simulink model "RobotControl"  (R2016a)
settings: Solver=FixedStepDiscrete  StartTime=0.0  StopTime=16  FixedStep=0.005  RelTol=1e-3
values from neighbouring files (symbols this model uses):
  BACKWARD = 2    [ControlInit.m]
  BUSY = 4    [ControlInit.m]
  CCW = 4    [ControlInit.m]
  CLEANED = 2    [ControlInit.m]
  CW = 3    [ControlInit.m]
  EMPTY = 3    [ControlInit.m]
  FORWARD = 1    [ControlInit.m]
  GTSP = 25    [ControlInit.m]
  initX = uint8((ROOM_SIDE_SIZE/2) - 1)    [ControlInit.m]
  initY = initX    [ControlInit.m]
  LEFT_BUSY_RIGHT_BUSY = 9    [ControlInit.m]
  LEFT_BUSY_RIGHT_CLEANED = 14    [ControlInit.m]
  LEFT_BUSY_RIGHT_EMPTY = 7    [ControlInit.m]
  LEFT_CLEANED_RIGHT_BUSY = 13    [ControlInit.m]
  LEFT_CLEANED_RIGHT_CLEANED = 12    [ControlInit.m]
  LEFT_CLEANED_RIGHT_EMPTY = 10    [ControlInit.m]
  LEFT_EMPTY_RIGHT_BUSY = 8    [ControlInit.m]
  LEFT_EMPTY_RIGHT_CLEANED = 11    [ControlInit.m]
  LEFT_EMPTY_RIGHT_EMPTY = 15    [ControlInit.m]
  map = uint8(ones(ROOM_SIDE_SIZE , ROOM_SIDE_SIZE)*UNCOVERED)    [ControlInit.m]
  MOVE_TURN_LEFT = 20    [ControlInit.m]
  MOVE_TURN_RIGHT = 21    [ControlInit.m]
  MOVE_U_TURN = 24    [ControlInit.m]
  MOVE_U_TURN_LEFT = 23    [ControlInit.m]
  MOVE_U_TURN_RIGHT = 22    [ControlInit.m]
  ROB_EAST = 0    [ControlInit.m]
  ROB_ERRVAL = 5    [ControlInit.m]
  ROB_NONE = 400    [ControlInit.m]
  ROB_NORTH = 270    [ControlInit.m]
  ROB_SOUTH = 90    [ControlInit.m]
  ROB_WEST = 180    [ControlInit.m]
  ROOM_SIDE_SIZE = 20    [ControlInit.m]
  STOP = 5    [ControlInit.m]
  UNCOVERED = 1    [ControlInit.m]
  ZIGZAG = 26    [ControlInit.m]
undefined symbols (not defined in the file or in its folder): COMH, Compass_Handler, MovementHandler, MOVH, POSH, positionHandler, ROB_LENG, ROTH, Routines, SAMPLE_TIME
libraries: simulink x2, SCAN x1, MAPH x1, MOTH x1
(part 2 of 2)

== stateflow chart RobotControl/Routines/HitSensorViewCalculation/pumperHitSensorView ==
  state SensorViewState
  state Init
    entry:
    sensorView = 0;
  state NoHit
    entry:
    currentY = c_Y - 1;
    currentX = c_X - 1;
  (junction 10) -> SensorViewState [order 1] : [(map[currentY][currentX - 1] == BUSY) ...
      | && ( (map[currentY][currentX + 1] == EMPTY)...
      |  || (map[currentY][currentX+1] == UNCOVERED) )]...
      | /sensorView = LEFT_BUSY_RIGHT_EMPTY;
  (junction 10) -> SensorViewState [order 2] : [(map[currentY][currentX - 1] == CLEANED) ...
      | && ((map[currentY][currentX + 1] == EMPTY)...
      | || (map[currentY][currentX+1] == UNCOVERED))]
      | /{sensorView =  LEFT_CLEANED_RIGHT_EMPTY;}
  (junction 10) -> SensorViewState [order 3] : [((map[currentY][currentX - 1] == EMPTY) ...
      | || (map[currentY][currentX - 1] == UNCOVERED))...
      | && (map[currentY][currentX + 1] == BUSY)]
      | /{sensorView = LEFT_EMPTY_RIGHT_BUSY;}
  (junction 10) -> SensorViewState [order 4] : [(map[currentY][currentX + 1] == CLEANED) ...
      | && ((map[currentY][currentX - 1] == EMPTY)...
      | || (map[currentY][currentX - 1] == UNCOVERED))]
      | /{sensorView =  LEFT_EMPTY_RIGHT_CLEANED;}
  (junction 10) -> SensorViewState [order 5] : [((map[currentY][currentX + 1] == EMPTY) ...
      | || (map[currentY][currentX + 1] == UNCOVERED))...
      | && ((map[currentY][currentX - 1] == EMPTY)...
      | || (map[currentY][currentX - 1] == UNCOVERED))]
      | /{sensorView = LEFT_EMPTY_RIGHT_EMPTY;}
  (junction 10) -> SensorViewState [order 6] : [(map[currentY][currentX - 1] == BUSY) ...
      | && (map[currentY][currentX + 1] == BUSY)]
      | /{sensorView = LEFT_BUSY_RIGHT_BUSY;}
  (junction 10) -> SensorViewState [order 7] : [(map[currentY][currentX - 1] == CLEANED) ...
      | && (map[currentY][currentX + 1] == CLEANED)]
      | /{sensorView = LEFT_CLEANED_RIGHT_CLEANED;}
  (junction 10) -> SensorViewState [order 8] : [(map[currentY][currentX - 1] == BUSY) ...
      | && (map[currentY][currentX + 1] == CLEANED)]
      | /{sensorView = LEFT_BUSY_RIGHT_CLEANED;}
  (junction 10) -> SensorViewState [order 9] : [(map[currentY][currentX - 1] == CLEANED) ...
      | && (map[currentY][currentX + 1] == BUSY)]
      | /{sensorView = LEFT_CLEANED_RIGHT_BUSY;}
  (junction 8) -> (junction 10) [order 1] : [currentHeading == ROB_NORTH]
  (default) -> Init
  (junction 11) -> SensorViewState [order 2] : [(map[currentY][currentX - 1] == BUSY) ...
      | && ( (map[currentY][currentX + 1] == EMPTY)...
      |  || (map[currentY][currentX+1] == UNCOVERED) )]...
      | /sensorView = LEFT_EMPTY_RIGHT_BUSY;
  Init -> NoHit
  NoHit -> (junction 8) : [pumperHit_BOOL]
  (junction 8) -> (junction 15) [order 4] : [currentHeading == ROB_EAST]
  (junction 8) -> (junction 13) [order 3] : [currentHeading == ROB_WEST]
  (junction 8) -> (junction 11) [order 2] : [currentHeading == ROB_SOUTH]
  SensorViewState -> NoHit
  (junction 11) -> SensorViewState [order 1] : [(map[currentY][currentX - 1] == CLEANED) ...
      | && ((map[currentY][currentX + 1] == EMPTY)...
      | || (map[currentY][currentX+1] == UNCOVERED))]
      | /{sensorView =  LEFT_EMPTY_RIGHT_CLEANED;}
  (junction 11) -> SensorViewState [order 5] : [((map[currentY][currentX - 1] == EMPTY) ...
      | || (map[currentY][currentX - 1] == UNCOVERED))...
      | && (map[currentY][currentX + 1] == BUSY)]
      | /{sensorView = LEFT_BUSY_RIGHT_EMPTY;}
  (junction 11) -> SensorViewState [order 6] : [(map[currentY][currentX + 1] == CLEANED) ...
      | && ((map[currentY][currentX - 1] == EMPTY)...
      | || (map[currentY][currentX - 1] == UNCOVERED))]
      | /{sensorView =  LEFT_CLEANED_RIGHT_EMPTY;}
  (junction 11) -> SensorViewState [order 4] : [((map[currentY][currentX + 1] == EMPTY) ...
      | || (map[currentY][currentX + 1] == UNCOVERED))...
      | && ((map[currentY][currentX - 1] == EMPTY)...
      | || (map[currentY][currentX - 1] == UNCOVERED))]
      | /{sensorView = LEFT_EMPTY_RIGHT_EMPTY;}
  (junction 11) -> SensorViewState [order 8] : [(map[currentY][currentX - 1] == BUSY) ...
      | && (map[currentY][currentX + 1] == CLEANED)]
      | /{sensorView = LEFT_CLEANED_RIGHT_BUSY;}
  (junction 11) -> SensorViewState [order 3] : [(map[currentY][currentX - 1] == BUSY) ...
      | && (map[currentY][currentX + 1] == BUSY)]
      | /{sensorView = LEFT_BUSY_RIGHT_BUSY;}
  (junction 11) -> SensorViewState [order 7] : [(map[currentY][currentX - 1] == CLEANED) ...
      | && (map[currentY][currentX + 1] == CLEANED)]
      | /{sensorView = LEFT_CLEANED_RIGHT_CLEANED;}
  (junction 11) -> SensorViewState [order 9] : [(map[currentY][currentX - 1] == CLEANED) ...
      | && (map[currentY][currentX + 1] == BUSY)]
      | /{sensorView = LEFT_BUSY_RIGHT_CLEANED;}
  data: c_X input; c_Y input; pumperHit_BOOL input; sensorView output uint8; map input size=[ROOM_SIDE_SIZE ROOM_SIDE_SIZE]; currentHeading input; BUSY input; EMPTY input; CLEANED input; UNCOVERED input; LEFT_BUSY_RIGHT_EMPTY input; LEFT_CLEANED_RIGHT_EMPTY input; LEFT_EMPTY_RIGHT_BUSY input; LEFT_EMPTY_RIGHT_CLEANED input; LEFT_EMPTY_RIGHT_EMPTY input; LEFT_BUSY_RIGHT_BUSY input; LEFT_CLEANED_RIGHT_CLEANED input; LEFT_BUSY_RIGHT_CLEANED input; LEFT_CLEANED_RIGHT_BUSY input; ROB_NORTH input; ROB_SOUTH input; ROB_WEST input; ROB_EAST input; currentX local uint8; currentY local uint8

== stateflow chart RobotControl/Routines/RoutineControl/Chart ==
  state GTSP
    entry:
    currentRoutine = GTSP;
  state init
  state ZIGZAG
    entry:
    currentRoutine = ZIGZAG;
  state End
  (default) -> init
  GTSP -> ZIGZAG : [GT_active == false]
  init -> GTSP
  ZIGZAG -> End : [ZG_active == false]
  data: currentRoutine output uint8; GT_active input; ZG_active input; GTSP input; ZIGZAG input; counter local uint16

== stateflow chart RobotControl/Compass_Handler/HeadingCalculation ==
  state initializeDirection
    entry:
    offset = theta;
  state Calc
    entry:
    theta_OUT = theta;
    //remove for now - offset
  state CalcHeading
    (default) -> (junction 2)
    (junction 2) -> (junction 3) [order 1] : [(theta_OUT <= 270 + ROB_ERRVAL) && (theta_OUT >= 270 - ROB_ERRVAL)]//NORTH
    (junction 2) -> (junction 4) [order 2]
    (junction 3) -> (junction 17) : {currentHeading = ROB_NORTH;}
    (junction 4) -> (junction 5) [order 1] : [(theta_OUT <= 90 + ROB_ERRVAL) && (theta_OUT >= 90 - ROB_ERRVAL)]//SOUTH
    (junction 4) -> (junction 6) [order 2]
    (junction 5) -> (junction 16) : {currentHeading = ROB_SOUTH;}
    (junction 6) -> (junction 7) [order 1] : [(theta_OUT <= 0 + ROB_ERRVAL) || (theta_OUT >= 360 - ROB_ERRVAL)]//EAST
    (junction 6) -> (junction 8) [order 2]
    (junction 7) -> (junction 15) : {currentHeading = ROB_EAST;}
    (junction 8) -> (junction 9) [order 1] : [(theta_OUT <= 180 + ROB_ERRVAL) && (theta_OUT >= 180 - ROB_ERRVAL)]//WEST
    (junction 8) -> (junction 12) [order 2] : {currentHeading = ROB_NONE;}
    (junction 9) -> (junction 14) : {currentHeading = ROB_WEST;}
    (junction 14) -> (junction 12)
    (junction 15) -> (junction 14)
    (junction 16) -> (junction 15)
    (junction 17) -> (junction 16)
    (junction 12) -> (junction 18)
  Calc -> CalcHeading [order 3]
  (default) -> initializeDirection
  initializeDirection -> Calc
  Calc -> (junction 54) [order 1] : [theta_OUT < 0]
  (junction 54) -> CalcHeading : /theta_OUT = theta_OUT + 360;
  CalcHeading -> Calc : [hasChanged(theta)]
  Calc -> (junction 57) [order 2] : [theta_OUT < ROB_ERRVAL]
  (junction 57) -> CalcHeading : /theta_OUT = ROB_ERRVAL;
  data: theta input; ROB_NORTH input; ROB_SOUTH input; ROB_WEST input; ROB_EAST input; ROB_NONE input; ROB_ERRVAL input; theta_OUT local int16; currentHeading output uint16; offset local int16

== stateflow chart RobotControl/positionHandler/positionUpdate ==
  state init
    en:
    currentY = initY;
    currentX = initX;
  state inMove
  state North
  state West
  state South
  state East
  (default) -> init
  init -> inMove
  (junction 52) -> inMove
  (junction 15) -> inMove [order 1] : [(((currentY + 1) >=...
      |  ROOM_SIDE_SIZE)...
      | && (turnRequest == BACKWARD))...
      | ||...
      | (((currentY - 1) <= 0)...
      | &&(turnRequest == FORWARD))]
      | /posStopReq = true;
  (junction 24) -> inMove [order 1] : [(((currentX + 1) >=...
      |  ROOM_SIDE_SIZE)...
      | && (turnRequest == BACKWARD))...
      | ||...
      | (((currentX - 1) <= 0)...
      | &&(turnRequest == FORWARD))]
      | /posStopReq = true;
  inMove -> (junction 13) : [(completedStep == true)...
      | && hasChanged(completedStep)]
      | /posStopReq = false;
  (junction 30) -> inMove [order 1] : [(((currentY + 1) >=...
      |  ROOM_SIDE_SIZE)...
      | &&(turnRequest == FORWARD))...
      | ||...
      | (((currentY - 1) <= 0)...
      | && (turnRequest == BACKWARD))]
      | /posStopReq = true;
  (junction 36) -> inMove [order 1] : [(((currentX + 1) >=...
      |  ROOM_SIDE_SIZE)...
      | &&(turnRequest == FORWARD))...
      | ||...
      | (((currentX - 1) <= 0)...
      | && (turnRequest == BACKWARD))]
      | /posStopReq = true;
  (junction 13) -> (junction 36) [order 4] : [currentHeading == ROB_EAST]
  (junction 13) -> (junction 15) [order 1] : [currentHeading == ROB_NORTH]
  (junction 13) -> (junction 30) [order 3] : [currentHeading == ROB_SOUTH]
  (junction 13) -> (junction 24) [order 2] : [currentHeading == ROB_WEST]
  (junction 15) -> North [order 2] : [(turnRequest == FORWARD)]
      | /currentY--;
  (junction 15) -> North [order 3] : [turnRequest == BACKWARD]
      | /currentY++;
  (junction 24) -> West [order 2] : [turnRequest == FORWARD]
      | /currentX--;
  (junction 30) -> South [order 3] : [turnRequest == BACKWARD]
      | /currentY--;
  (junction 30) -> South [order 2] : [turnRequest == FORWARD]
      | /currentY++;
  (junction 36) -> East [order 2] : [turnRequest == FORWARD]
      | /currentX++;
  (junction 24) -> West [order 3] : [turnRequest == BACKWARD]
      | /currentX++;
  (junction 36) -> East [order 3] : [turnRequest == BACKWARD]
      | /currentX--;
  East -> (junction 52)
  North -> (junction 52)
  West -> (junction 52)
  South -> (junction 52)
  data: ROB_EAST input; ROB_NORTH input; ROB_SOUTH input; ROB_WEST input; currentX output uint8; currentY output uint8; initX input; initY input; completedStep input; currentHeading input; turnRequest input; BACKWARD input; FORWARD input; posStopReq output boolean; ROOM_SIDE_SIZE input

== stateflow chart RobotControl/Routines/zigzagRoutine/Chart ==
  state SwitchLane
  state finishZigZag
    en:
    zgzgActive = false;
    moveRequest = STOP;
  state Idle
  state MovingForward
    en:
    moveRequest = FORWARD;
  (junction 34) -> SwitchLane [order 1] : [currentHeading == ROB_NORTH]
      | /moveRequest = MOVE_U_TURN_RIGHT;
      | headingRequest = ROB_SOUTH;
  (junction 34) -> SwitchLane [order 2] : [currentHeading == ROB_SOUTH]
      | /moveRequest = MOVE_U_TURN_LEFT;
      | headingRequest = ROB_NORTH;
  (junction 35) -> SwitchLane [order 1] : [currentHeading == ROB_NORTH]
      | /moveRequest = MOVE_U_TURN_RIGHT;
      | headingRequest = ROB_SOUTH;
  (junction 33) -> (junction 34) [order 1] : [sensorView == LEFT_EMPTY_RIGHT_EMPTY]
  SwitchLane -> finishZigZag [order 1] : [finishCounter > 2]
  (junction 35) -> SwitchLane [order 2] : [currentHeading == ROB_SOUTH]
      | /moveRequest = MOVE_U_TURN;
      | headingRequest = ROB_NORTH;
  (junction 33) -> (junction 35) [order 2] : [(sensorView == LEFT_CLEANED_RIGHT_EMPTY)...
      | || (sensorView == LEFT_BUSY_RIGHT_EMPTY)]
  (junction 36) -> SwitchLane [order 2] : [currentHeading == ROB_SOUTH]
      | /moveRequest = MOVE_U_TURN_LEFT;
      | headingRequest = ROB_NORTH;
  (default) -> Idle
  Idle -> MovingForward : [currentRoutine == ZIGZAG]
      | /zgzgActive = true;
  MovingForward -> (junction 33) : [pumperInterrupt_BOOL]
      | /moveRequest = STOP;
  (junction 36) -> SwitchLane [order 1] : [currentHeading == ROB_NORTH]
      | /moveRequest = MOVE_U_TURN;
      | headingRequest = ROB_SOUTH;
  (junction 33) -> (junction 36) [order 3] : [(sensorView == LEFT_EMPTY_RIGHT_CLEANED)...
      | || (sensorView == LEFT_EMPTY_RIGHT_BUSY)]
  (junction 33) -> (junction 37) [order 4] : [(sensorView == LEFT_BUSY_RIGHT_BUSY)...
      | || (sensorView == LEFT_BUSY_RIGHT_CLEANED)...
      | || (sensorView == LEFT_CLEANED_RIGHT_BUSY)...
      | || (sensorView == LEFT_CLEANED_RIGHT_CLEANED)]
  SwitchLane -> MovingForward [order 2] : [(headingRequest == currentHeading)...
      | && (targetReached == true)]
  (junction 37) -> SwitchLane [order 1] : [currentHeading == ROB_NORTH]
      | /moveRequest = MOVE_U_TURN;
      | headingRequest = ROB_SOUTH;
      | finishCounter++;
  (junction 37) -> SwitchLane [order 2] : [currentHeading == ROB_SOUTH]
      | /moveRequest = MOVE_U_TURN;
      | headingRequest = ROB_NORTH;
      | finishCounter++;
  data: LEFT_BUSY_RIGHT_EMPTY input; LEFT_CLEANED_RIGHT_EMPTY input; LEFT_EMPTY_RIGHT_BUSY input; LEFT_EMPTY_RIGHT_CLEANED input; LEFT_EMPTY_RIGHT_EMPTY input; LEFT_BUSY_RIGHT_BUSY input; LEFT_CLEANED_RIGHT_CLEANED input; LEFT_BUSY_RIGHT_CLEANED input; LEFT_CLEANED_RIGHT_BUSY input; ROB_NORTH input; ROB_SOUTH input; ROB_WEST input; ROB_EAST input; FORWARD input; MOVE_TURN_LEFT input; MOVE_TURN_RIGHT input; MOVE_U_TURN input; MOVE_U_TURN_RIGHT input; MOVE_U_TURN_LEFT input; sensorView input; STOP input; moveRequest output uint8; currentHeading input; currentRoutine input; pumperInterrupt_BOOL input; targetReached input; headingRequest local double; ZIGZAG parameter; zgzgActive output boolean =true;; finishCounter local uint8
